simulink model "model1"  (R2019b)
settings: Solver=VariableStepAuto  StartTime=0.0  StopTime=10.0  RelTol=1e-3
settings Model: Creator=surtweig  LastModifiedBy=surtweig

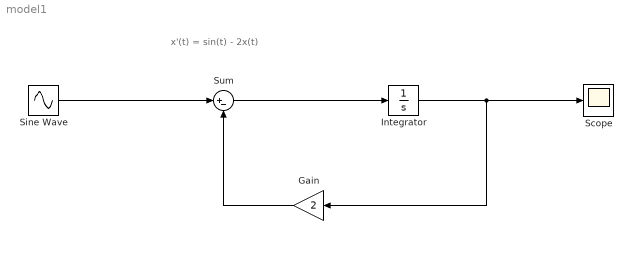
== system model1 ==
  note: x'(t) = sin(t) - 2x(t)
  Gain : Gain  Gain=2
  Integrator : Integrator
  Scope : Scope
  Sine Wave : Sin  SampleTime=0
  Sum : Sum  Inputs=|+-
  wires:
  Sum/1 -> Integrator/1
  Gain/1 -> Sum/2
  Integrator/1 -> Gain/1, Scope/1
  Sine Wave/1 -> Sum/1
